simulink model "linearizedPNG"  (Simulink 7.1)
settings: Solver=ode45  StartTime=0.0  StopTime=TFINAL-0.0001  RelTol=1e-3
values from neighbouring files (symbols this model uses):
  AT = 3    [linearizedPNG_ini.m]    (also in missdisatnce_adjoint.m; missdistance_homing_loop.m; missdistance_linearized.m; truePNG_ini.m = 0)
  HE = 0*(-30/180*pi)    (= 0)    [linearizedPNG_ini.m]    (also in missdisatnce_adjoint.m = 0.523598775598; missdistance_homing_loop.m; missdistance_linearized.m)
  MAX_ACC = 7    [linearizedPNG_ini.m]    (also in truePNG_ini.m = 0.5)
  Tautopilot = 0    [linearizedPNG_ini.m]    (also in missdisatnce_adjoint.m = 2; missdistance_homing_loop.m = 2; missdistance_linearized.m = 2; truePNG_ini.m = 0.2)
  TFINAL = 10    [linearizedPNG_ini.m]    (also in missdisatnce_adjoint.m = 20)
  VC = VM+VT    (= 140)    [linearizedPNG_ini.m]
  VM = 100    [linearizedPNG_ini.m]    (also in truePNG_ini.m = 0.5)
libraries: simulink x1
settings Model: Creator=LESSONS  LastModifiedBy=LESSONS
settings DebuggingCC: SolverPrmCheckMsg=none

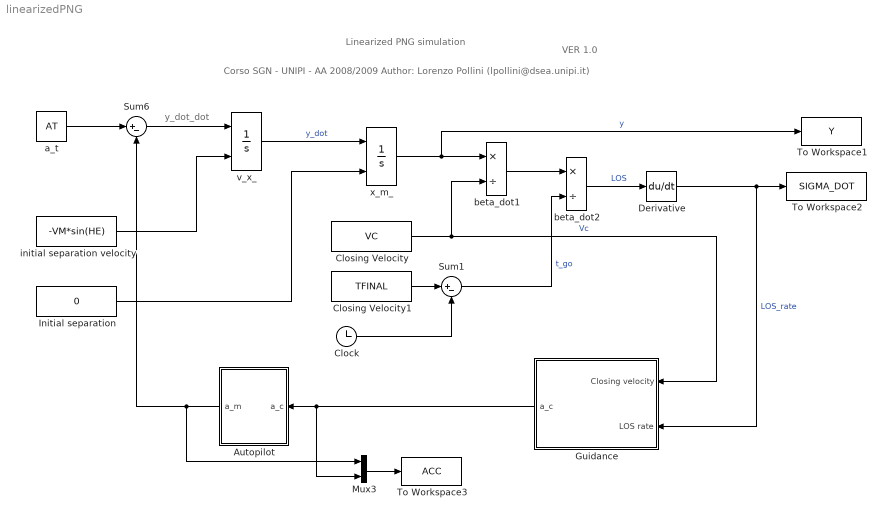
== system linearizedPNG ==
  note: y_dot_dot
  note: Linearized PNG simulation
  note: Corso SGN - UNIPI - AA 2008/2009
      | Author: Lorenzo Pollini (lpollini@dsea.unipi.it)
  note: VER 1.0
  Autopilot : Subsystem  Orientation=left
  Clock : Clock
      settings: Decimation=10
  Closing Velocity : Constant  Value=VC  OutDataType=sfix(16)  OutScaling=2^0
  Closing Velocity1 : Constant  Value=TFINAL  OutDataType=sfix(16)  OutScaling=2^0
  Derivative : Derivative
  Guidance : Subsystem  Orientation=left
  Initial separation : Constant  Value=0  OutDataType=sfix(16)  OutScaling=2^0
  Mux3 : Mux  Inputs=2
  Sum1 : Sum  Inputs=|+-  OutDataType=sfix(16)  OutScaling=2^0
  Sum6 : Sum  Inputs=|+-  OutDataType=sfix(16)  OutScaling=2^0
  To Workspace1 : ToWorkspace  VariableName=Y  SampleTime=-1  SaveFormat=Structure With Time
  To Workspace2 : ToWorkspace  VariableName=SIGMA_DOT  SampleTime=-1  SaveFormat=Structure With Time
  To Workspace3 : ToWorkspace  VariableName=ACC  SampleTime=-1  SaveFormat=Structure With Time
  a_t : Constant  Value=AT  OutDataType=sfix(16)  OutScaling=2^0
  beta_dot1 : Product  Inputs=*/  OutDataType=sfix(16)  OutScaling=2^-10
  beta_dot2 : Product  Inputs=*/  OutDataType=sfix(16)  OutScaling=2^-10
  initial separation velocity : Constant  Value=-VM*sin(HE)  OutDataType=sfix(16)  OutScaling=2^0
  v_x_ : Integrator  InitialConditionSource=external
  x_m_ : Integrator  InitialConditionSource=external
  wires:
  a_t/1 -> Sum6/1
  Guidance/1(a_c) -> Autopilot/1(a_c), Mux3/2
  Sum6/1 -> v_x_/1
  v_x_/1 -> x_m_/1  "y_dot"
  x_m_/1 -> beta_dot1/1, To Workspace1/1  "y"
  beta_dot1/1 -> beta_dot2/1
  Closing Velocity/1 -> beta_dot1/2, Guidance/1(Closing velocity)  "Vc"
  Closing Velocity1/1 -> Sum1/1
  Clock/1 -> Sum1/2
  Sum1/1 -> beta_dot2/2  "t_go"
  beta_dot2/1 -> Derivative/1  "LOS"
  Derivative/1 -> Guidance/2(LOS rate), To Workspace2/1  "LOS_rate"
  Autopilot/1(a_m) -> Sum6/2, Mux3/1
  initial separation velocity/1 -> v_x_/2
  Initial separation/1 -> x_m_/2
  Mux3/1 -> To Workspace3/1

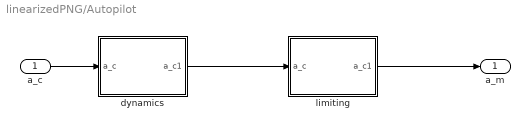
== system linearizedPNG/Autopilot ==
  a_c : Inport  OutDataType=sfix(16)  OutScaling=2^0
  dynamics : Subsystem
  limiting : Subsystem
  a_m : Outport  OutDataType=sfix(16)  OutScaling=2^0
  wires:
  a_c/1 -> dynamics/1(a_c)
  dynamics/1(a_c1) -> limiting/1(a_c)
  limiting/1(a_c1) -> a_m/1

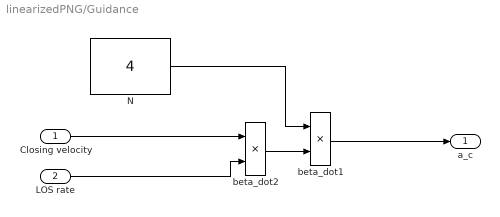
== system linearizedPNG/Guidance ==
  Closing velocity : Inport  OutDataType=sfix(16)  OutScaling=2^0
  LOS rate : Inport  Port=2  OutDataType=sfix(16)  OutScaling=2^0
  N : Constant  Value=4  OutDataType=sfix(16)  OutScaling=2^0
  beta_dot1 : Product  Inputs=**  OutDataType=sfix(16)  OutScaling=2^-10
  beta_dot2 : Product  Inputs=**  OutDataType=sfix(16)  OutScaling=2^-10
  a_c : Outport  OutDataType=sfix(16)  OutScaling=2^0
  wires:
  Closing velocity/1 -> beta_dot2/1
  beta_dot1/1 -> a_c/1
  LOS rate/1 -> beta_dot2/2
  beta_dot2/1 -> beta_dot1/2
  N/1 -> beta_dot1/1

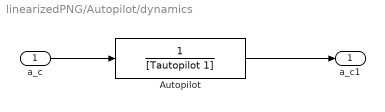
== system linearizedPNG/Autopilot/dynamics ==
  a_c : Inport  OutDataType=sfix(16)  OutScaling=2^0
  Autopilot : TransferFcn  Denominator=[Tautopilot 1]
  a_c1 : Outport  OutDataType=sfix(16)  OutScaling=2^0
  wires:
  a_c/1 -> Autopilot/1
  Autopilot/1 -> a_c1/1

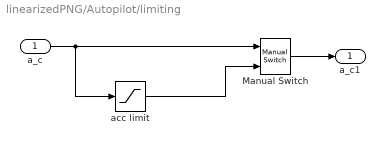
== system linearizedPNG/Autopilot/limiting ==
  a_c : Inport  OutDataType=sfix(16)  OutScaling=2^0
  Manual Switch : simulink/Signal Routing/Manual Switch  SystemSampleTime=-1  sw=1  action=0  varsize=off
  acc limit : Saturate  UpperLimit=MAX_ACC  LowerLimit=-MAX_ACC
  a_c1 : Outport  OutDataType=sfix(16)  OutScaling=2^0
  wires:
  Manual Switch/1 -> a_c1/1
  a_c/1 -> Manual Switch/1, acc limit/1
  acc limit/1 -> Manual Switch/2
